simulink model "dev_lab6"  (R2015b)
settings: Solver=ode3  StartTime=0  StopTime=10  FixedStep=Ts  RelTol=1e-3
values from neighbouring files (symbols this model uses):
  Ac = 5    [dev_digicomm_lab6.m]
  ph0 = -25*pi/180    (= -0.436332312999)    [dev_digicomm_lab6.m]
  ph1 = 50*pi/180    (= 0.872664625997)    [dev_digicomm_lab6.m]
  rc = fc*2*pi    (= 125663.706144)    [dev_digicomm_lab6.m]
  Tb = 1/rb    (= 0.001)    [dev_digicomm_lab6.m]
  Ts = Tb/500    (= 2e-06)    [dev_digicomm_lab6.m]
libraries: commfilt2 x1, commchan3 x1, commsink2 x1, commrandsrc2 x1
settings Model: Creator=Dennis Silage  LastModifiedBy=trejo
settings DataIOCC: SaveFormat=Array  SignalLoggingSaveFormat=ModelDataLogs
settings OptimizationCC: ExpressionDepthLimit=2147483647  InitFltsAndDblsToZero=on
settings DebuggingCC: UnderspecifiedInitializationDetection=Classic  MergeDetectMultiDrivingBlocksExec=none  SolverPrmCheckMsg=warning  FcnCallInpInsideContextMsg=UseLocalSettings  StateNameClashWarn=warning
settings HardwareCC: ProdBitPerPointer=32  ProdLargestAtomicFloat=None  ProdIntDivRoundTo=Undefined  ProdEndianess=Unspecified  ProdWordSize=32  ProdHWDeviceType=32-bit Generic
settings GRTTargetCC: GeneratePreprocessorConditionals=Disable all  CombineOutputUpdateFcns=off  GRTInterface=on
settings ConfigComp: CovModelRefEnable=Off  CovSFcnEnable=off

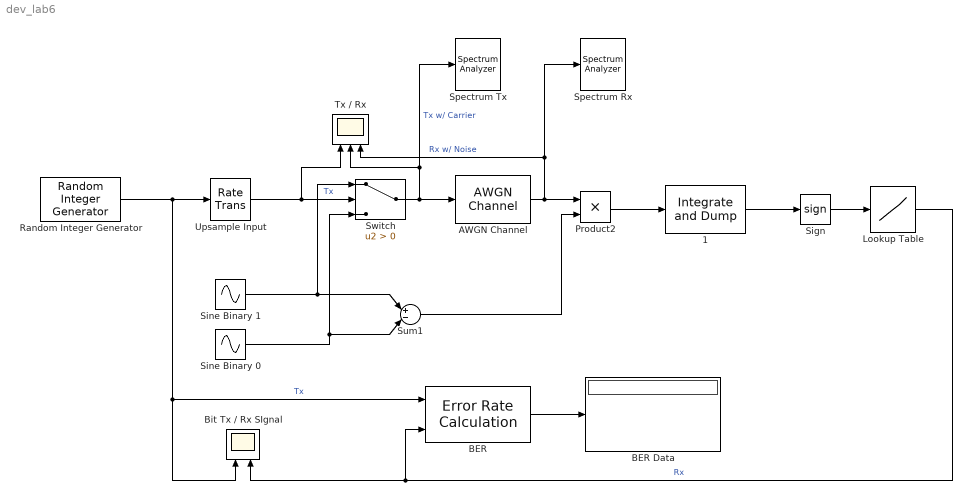
== system dev_lab6 ==
  " 1" : commfilt2/Integrate and Dump  obssamples=intT  offsetsamples=0  nodump=off  roundingMode=Floor  overflowMode=off
  AWGN Channel : commchan3/AWGN Channel  InputProcessing=Columns as channels (frame based)  seed=randseed  noiseMode=Variance from mask  EbNodB=90  EsNodB=10  SNRdB=10  bitsPerSym=1  Ps=25  Tsym=1e-3  variance=N0
  BER : commsink2/Error Rate Calculation  N=2  st_delay=0  cp_mode=Entire frame  subframe=[]  PMode=Port  WsName=ErrorVec  RsMode2=off  stop=off  numErr=100  maxBits=1e6
  BER Data : Display
  Bit Tx / Rx SIgnal : Scope  NumInputPorts=2
  Lookup Table : Lookup  InputValues=[-1,0,1]  Table=[0,0,1]
  Product2 : Product
  Random Integer Generator : commrandsrc2/Random Integer Generator  mul=2  seed=randseed  Ts=Tb  frameBased=off  sampPerFrame=1  orient=on  outDataType=double
  Sign : Signum
  Sine Binary 0 : Sin  Amplitude=Ac  Frequency=rc  Phase=ph0  SampleTime=Ts
  Sine Binary 1 : Sin  Amplitude=Ac  Frequency=rc  Phase=ph1  SampleTime=Ts
  Spectrum Rx : SpectrumAnalyzer
  Spectrum Tx : SpectrumAnalyzer
  Sum1 : Sum  Inputs=|+-|
  Switch : Switch  Criteria=u2 > Threshold
  Tx / Rx : Scope  NumInputPorts=3
  Upsample Input : RateTransition  OutPortSampleTime=Ts
  wires:
  BER/1 -> BER Data/1
  Switch/1 -> AWGN Channel/1, Tx / Rx/2, Spectrum Tx/1  "Tx w/ Carrier"
  Random Integer Generator/1 -> BER/1, Bit Tx / Rx SIgnal/1, Upsample Input/1  "Tx"
  Upsample Input/1 -> Tx / Rx/1, Switch/2  "Tx"
  Sign/1 -> Lookup Table/1
  " 1"/1 -> Sign/1
  Product2/1 -> " 1"/1
  Lookup Table/1 -> BER/2, Bit Tx / Rx SIgnal/2  "Rx"
  AWGN Channel/1 -> Product2/1, Tx / Rx/3, Spectrum Rx/1  "Rx w/ Noise"
  Sum1/1 -> Product2/2
  Sine Binary 0/1 -> Switch/3, Sum1/2
  Sine Binary 1/1 -> Sum1/1, Switch/1
